simulink model "inbuiltNavigation"  (R2021b)
settings: Solver=VariableStepAuto  StartTime=0.0  StopTime=inf  FixedStep=0.001  RelTol=1e-3
model workspace (MAT data in the model file):
  enableTransmit = 1
libraries: mspfiltlib x1, sensorgpslib x1, instrumentlib x1, mspsensorlib x1, sensorinslib x1
settings Model: Creator=Vladik  LastModifiedBy=Vladik

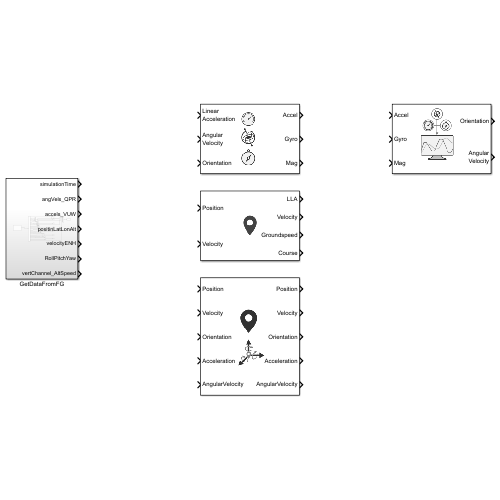
[thumbnail: Simulink's stored preview of the top-level diagram]
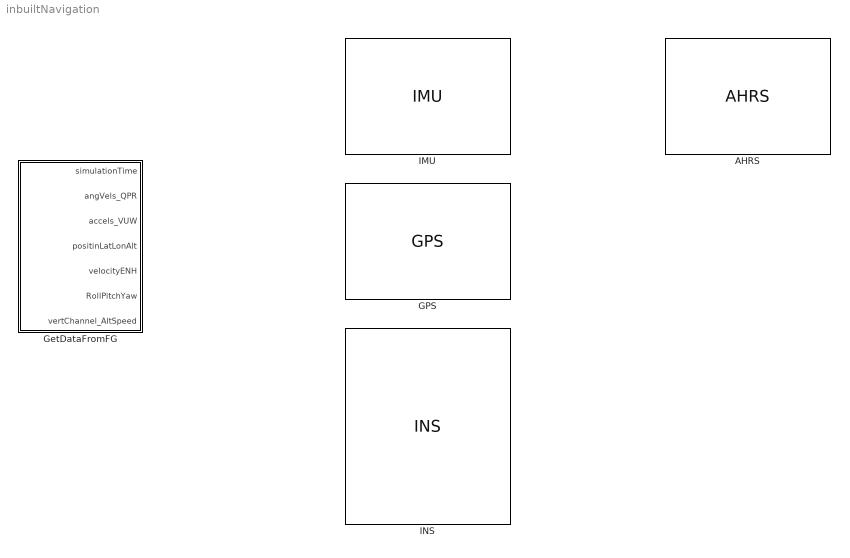
== system inbuiltNavigation ==
  AHRS : mspfiltlib/AHRS  DispRefFrame=NED  DecimationFactor=1  InitialProcessNoise=ahrsfilter.defaultProcessNoise  OrientationFormat=quaternion  SimulateUsing=Interpreted execution  AccelerometerNoise=0.0001924722  GyroscopeNoise=9.1385e-5  MagnetometerNoise=0.1  GyroscopeDriftNoise=3.0462e-13  LinearAccelerationNoise=0.0096236100000000012  MagneticDisturbanceNoise=0.5  LinearAccelerationDecayFactor=0.5  MagneticDisturbanceDecayFactor=0.5  ExpectedMagneticFieldStrength=50
      settings: SourceProductBaseCode=TF,NV
  GPS : sensorgpslib/GPS  DispRefFrame=NED  PositionInputFormat=Local  ReferenceLocation=[ 0, 0, 0 ]  HorizontalPositionAccuracy=1.6  VerticalPositionAccuracy=3  VelocityAccuracy=0.1  DecayFactor=0.999  SeedDouble=67  SimulateUsing=Interpreted execution
      settings: SourceProductBaseCode=TF,NV,UV
  GetDataFromFG : Subsystem
  IMU : mspsensorlib/IMU  DispRefFrame=NED  Temperature=25  MagneticFieldNED=[ 27.5550, -2.4169, -16.0849 ]  MagneticFieldENU=[ -2.4169, 27.5550, 16.0849 ]  SeedDouble=67  SimulateUsing=Interpreted execution  AccelParamsMeasurementRange=Inf  AccelParamsResolution=0  AccelParamsConstantBias=[ 0, 0, 0 ]  AccelParamsAxesMisalignment=[ 100, 0, 0; 0, 100, 0; 0, 0, 100 ]  AccelParamsNoiseDensity=[ 0, 0, 0 ]  AccelParamsBiasInstability=[ 0, 0, 0 ]  AccelParamsRandomWalk=[ 0, 0, 0 ]  AccelParamsTemperatureBias=[ 0, 0, 0 ]  AccelParamsTemperatureScaleFactor=[ 0, 0, 0 ]  GyroParamsMeasurementRange=Inf  GyroParamsResolution=0  GyroParamsConstantBias=[ 0, 0, 0 ]  GyroParamsAxesMisalignment=[ 100, 0, 0; 0, 100, 0; 0, 0, 100 ]  GyroParamsAccelerationBias=[ 0, 0, 0 ]  GyroParamsNoiseDensity=[ 0, 0, 0 ]  GyroParamsBiasInstability=[ 0, 0, 0 ]  GyroParamsRandomWalk=[ 0, 0, 0 ]  GyroParamsTemperatureBias=[ 0, 0, 0 ]  GyroParamsTemperatureScaleFactor=[ 0, 0, 0 ]  MagParamsMeasurementRange=Inf  MagParamsResolution=0  MagParamsConstantBias=[ 0, 0, 0 ]  MagParamsAxesMisalignment=[ 100, 0, 0; 0, 100, 0; 0, 0, 100 ]  MagParamsNoiseDensity=[ 0, 0, 0 ]  MagParamsBiasInstability=[ 0, 0, 0 ]  MagParamsRandomWalk=[ 0, 0, 0 ]  MagParamsTemperatureBias=[ 0, 0, 0 ]  MagParamsTemperatureScaleFactor=[ 0, 0, 0 ]
      settings: SourceProductBaseCode=TF,NV
  INS : sensorinslib/INS  MountingLocation=[0 0 0]  RollAccuracy=0.2  PitchAccuracy=0.2  YawAccuracy=1  PositionAccuracy=1  VelocityAccuracy=0.05  UseAccelAndAngVel=on  AccelerationAccuracy=0  AngularVelocityAccuracy=0  TimeInput=off  PositionErrorFactor=[0 0 0]  SeedDouble=67  SimulateUsing=Code generation
      settings: SourceProductBaseCode=DR,TF,NV,UV

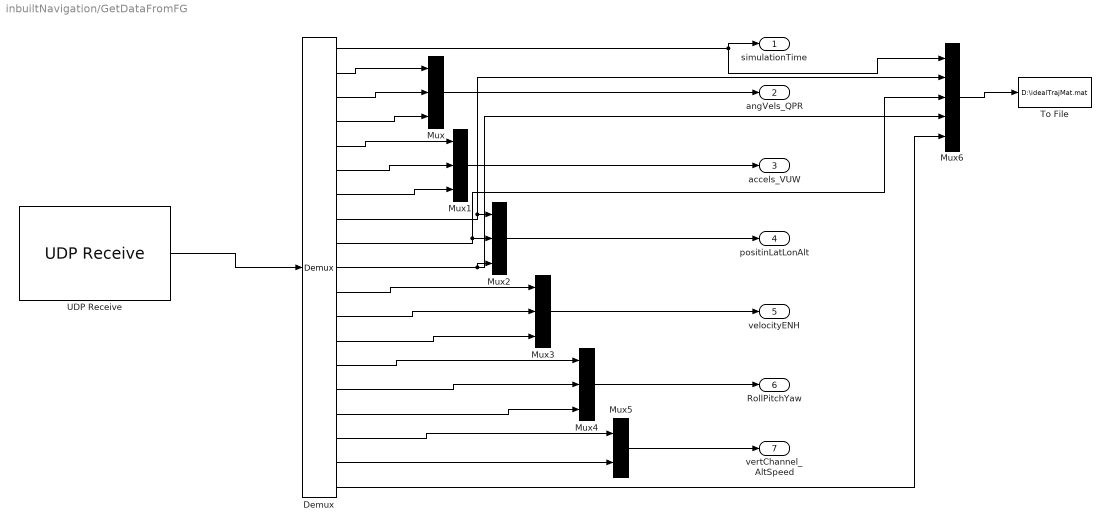
== system inbuiltNavigation/GetDataFromFG ==
  Demux : Demux  Outputs=19
  Mux{,1..4} (5 alike) : Mux  Inputs=3
  Mux5 : Mux  Inputs=2
  Mux6 : Mux  Inputs=5
  To File : ToFile  Filename=D:\idealTrajMat.mat  MatrixName=idealTrajData
  UDP Receive : instrumentlib/UDP Receive  Host=localhost  Port=10000  LocalPort=10000  EnablePortSharing=off  GetLatestData=off  DataSize="[1  19]"  DataType=ASCII  ASCIIFormatting=%f %f %f %f %f %f %f %f %f %f %f %f %f %f %f %f %f %f %f  Terminator=LF  ByteOrder=BigEndian  EnableBlockingMode=on  Timeout=10  SampleTime=0.01  LocalAddress=localhost
  simulationTime : Outport
  angVels_QPR : Outport  Port=2
  accels_VUW : Outport  Port=3
  positinLatLonAlt : Outport  Port=4
  velocityENH : Outport  Port=5
  RollPitchYaw : Outport  Port=6
  vertChannel_AltSpeed : Outport  Port=7
  wires:
  UDP Receive/1 -> Demux/1
  Demux/2 -> Mux/1
  Demux/3 -> Mux/2
  Demux/4 -> Mux/3
  Demux/5 -> Mux1/1
  Demux/6 -> Mux1/2
  Demux/7 -> Mux1/3
  Demux/8 -> Mux6/2, Mux2/1
  Demux/9 -> Mux6/3, Mux2/2
  Demux/10 -> Mux2/3, Mux6/4
  Mux/1 -> angVels_QPR/1
  Mux1/1 -> accels_VUW/1
  Mux2/1 -> positinLatLonAlt/1
  Demux/11 -> Mux3/1
  Demux/12 -> Mux3/2
  Demux/13 -> Mux3/3
  Mux3/1 -> velocityENH/1
  Demux/14 -> Mux4/1
  Demux/15 -> Mux4/2
  Demux/16 -> Mux4/3
  Mux4/1 -> RollPitchYaw/1
  Demux/17 -> Mux5/1
  Demux/18 -> Mux5/2
  Mux5/1 -> vertChannel_AltSpeed/1
  Demux/1 -> simulationTime/1, Mux6/1
  Mux6/1 -> To File/1
  Demux/19 -> Mux6/5
